simulink model "FM_SDR_Receiver_PLL_Detector"  (R2022a)
settings: Solver=FixedStepDiscrete  StartTime=0.0  StopTime=inf  RelTol=1e-3
PreLoadFcn:
  | addpath('matlab/demodulation');
libraries: dspsigops x3, dspsnks4 x1, dsparch4 x1, sdrrlib x1
settings Model: Creator=Kate  LastModifiedBy=vovan
settings SolverCC: AlgebraicLoopSolver=TrustRegion
settings DebuggingCC: UnconnectedInputMsg=warning  UnconnectedOutputMsg=warning  UnconnectedLineMsg=warning  SFMachineParentedDataDiag=warning
settings SFSimCC: CustomCodeUndefinedFunction=UseInterfaceOnly

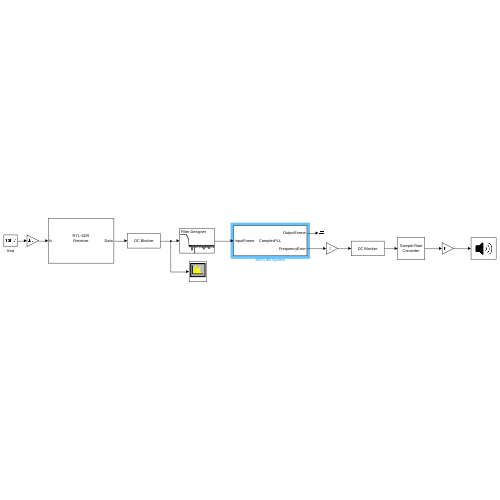
[thumbnail: Simulink's stored preview of the top-level diagram]
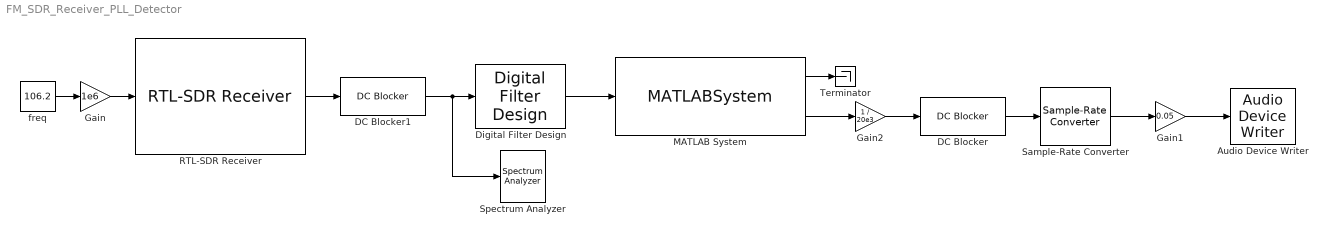
== system FM_SDR_Receiver_PLL_Detector ==
  Audio Device Writer : dspsnks4/Audio Device Writer  Driver=ALSA  Device=Default  InheritSampleRate=on  SampleRate=44100  BitDepth=16-bit integer  BufferSize=4096  NumBuffers=10  DefaultOutputChannelMapping=on  OutputChannelMapping=1:2  OutputNumUnderrunSamples=off  DriverIdx=8  DeviceWarnFlag=''
  DC Blocker : dspsigops/DC Blocker  Algorithm=IIR  NormalizedBandwidth=0.001  Length=50  Order=6  SimulateUsing=Code generation
      settings: SourceProductBaseCode=DS
  DC Blocker1 : dspsigops/DC Blocker  Algorithm=IIR  NormalizedBandwidth=0.001  Length=50  Order=6  SimulateUsing=Code generation
      settings: SourceProductBaseCode=DS
  Digital Filter Design : dsparch4/Digital Filter Design  mwdsp_browser_bugfix_var=off
  Gain : Gain  Gain=1e6
  Gain1 : Gain  Gain=0.05
  Gain2 : Gain  Gain=1 / 20e3
  MATLAB System : MATLABSystem  System=ComplexPLL  SampleFrequency=1.2e6  NoiseBandwidth=64e3  Dampingfactor=0.7  CentralFrequency=0  SimulateUsing=Code generation
      mask Type: ComplexPLL
      mask Display:
      | disp('ComplexPLL');
      | port_label('input',1,'InputFrame');
      | port_label('output',1,'OutputFrame');
      | port_label('output',2,'FrequencyError');
  RTL-SDR Receiver : sdrrlib/RTL-SDR Receiver  IPAddress=0  CenterFrequencySource=Input port  CenterFrequency=102.5e6  GainSource=AGC  Gain=0  ADCRate=1.2e6  FrequencyCorrection=0  LostSamplesOutputPort=off  LatencyOutputPort=off  OutputDataType=double  FrameLength=512*25  EnableBurstMode=off  NumFramesInBurst=20  sobjType=sdrr.internal.SDRRTLReceiverSL  dataUDPPort=-1  ctrlUDPPort=-1  subDeviceList=nosubdev  sdrBlockType=SDRBlockTypeSLT.SDRRxBlock  requester=UNUSED_BY_SFCN  sdrExecutionMode=SDRExecutionModeSLT.ExecModeHW  BypassUserLogic=off  DecimatorSelect=DDC decimator  SourceSelect=RF data  SineAmplitude=16000  EnableInternalClock=off  BypassIQBalance=off  IFBandwidth=40e6  ADCRateSource=Dialog  IntermediateFrequency=0  DecimationFactorSource=Dialog  DecimationFactor=512  RFFrequencyIsTunable=logical(1)  SampleTime=(512*25)/(1.2e6)  IFBandwidthSource=Dialog  SineFrequency=30000  BypassDCBlockingFilter=off  IntermediateFrequencySource=Dialog  IQBalanceCoefficients=64  SkipAllHardwareResetAndInitialization=off  EnableIQCalibrationTable=on  CacheIQCalibrationTable=off  EnableOffsetTuning=off  EnableRTLAGC=off  EnableTestMode=off  EnableTunerAGC=on  FrequencyCorrectionSource=Dialog  NumMLBuffers=128  NumUSBBuffers=16  RTLCrystalFrequency=28800000  TunerCrystalFrequency=28800000
      settings: SourceProductBaseCode=RTLSDR
  Sample-Rate Converter : dspsigops/Sample-Rate Converter  InputSampleRate=1.2e6  OutputSampleRate=48e3  OutputRateTolerance=0  Bandwidth=30e3  StopbandAttenuation=80  SimulateUsing=Code generation
      settings: SourceProductBaseCode=DS
  Spectrum Analyzer : SpectrumAnalyzer
  Terminator : Terminator
  freq : Constant  Value=106.2
  wires:
  freq/1 -> Gain/1
  Gain/1 -> RTL-SDR Receiver/1
  Sample-Rate Converter/1 -> Gain1/1
  RTL-SDR Receiver/1 -> DC Blocker1/1
  DC Blocker1/1 -> Spectrum Analyzer/1, Digital Filter Design/1
  DC Blocker/1 -> Sample-Rate Converter/1
  Digital Filter Design/1 -> MATLAB System/1
  MATLAB System/1 -> Terminator/1
  MATLAB System/2 -> Gain2/1
  Gain2/1 -> DC Blocker/1
  Gain1/1 -> Audio Device Writer/1
